simulink model "gm_sampleModel1427_5_sub"  (R2023a)
settings: Solver=VariableStepAuto  StartTime=0.0  StopTime=10.0  RelTol=1e-3
libraries: simulink x3
settings Model: Creator=user1  LastModifiedBy=user1
settings OptimizationCC: BlockReduction=off  ConditionallyExecuteInputs=off
settings DebuggingCC: InheritedTsInSrcMsg=none

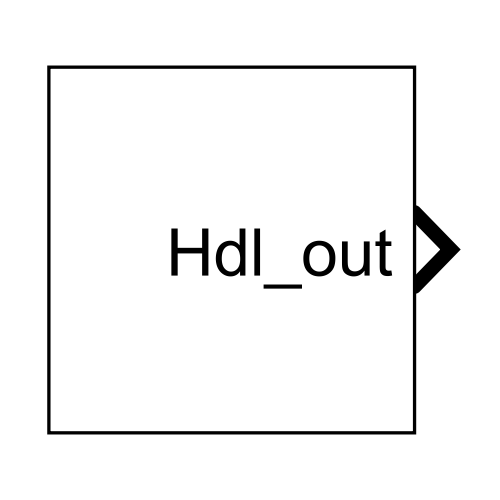
[thumbnail: Simulink's stored preview of the top-level diagram]
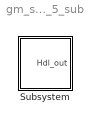
== system gm_sampleModel1427_5_sub ==
  Subsystem : Subsystem

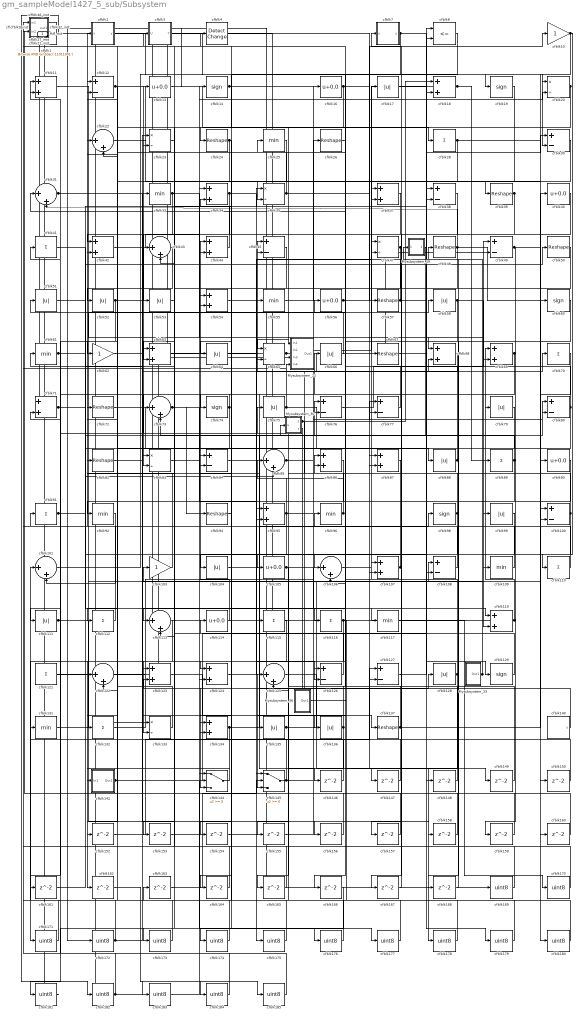
== system gm_sampleModel1427_5_sub/Subsystem ==
  Mysubsystem_19 : Subsystem
  Mysubsystem_22 : Subsystem
  Mysubsystem_30 : Subsystem
  Mysubsystem_33 : Subsystem
  Mysubsystem_36 : Subsystem
  cfblk1 : simulink/Logic and Bit Operations/Bitwise Operator  logicop=AND  UseBitMask=on  BitMask=bin2dec('11011001')  BitMaskRealWorld=Stored Integer
      settings: LibrarySourceBlock=|
      | hdlsllib/Logic and Bit
      | Operations/Bitwise
      | Operator
  cfblk10 : Gain  OutDataTypeStr=uint8
  cfblk{12,30,38,45,49,76..77,80,84,100,108,126..127} (13 alike) : Sum  Inputs=+-  OutDataTypeStr=uint8
  cfblk{22,31,43,73,85,101,106,113,122,125} (10 alike) : Sum  Inputs=|++  OutDataTypeStr=uint8
  cfblk102_inst : Subsystem
  cfblk103 : Gain  OutDataTypeStr=uint8
  cfblk{17,51..53,58,64,66,75,79,88,99,104,111,128,135..136} (16 alike) : Abs  OutDataTypeStr=uint8  SaturateOnIntegerOverflow=off
  cfblk{13,16,40,56,90,105,114} (7 alike) : Bias  Bias=0.0  SaturateOnIntegerOverflow=off
  cfblk{11,18,34,37,42,44,54,63,68..69,71,86..87,95,107,119,123..124,134} (19 alike) : Sum  OutDataTypeStr=uint8
  cfblk{25,33,55,61,92,96,109,117,131} (9 alike) : MinMax  OutDataTypeStr=uint8
  cfblk{28,41,70,89,91,110,112,115..116,121,132} (11 alike) : Sum  Inputs=+  OutDataTypeStr=uint8
  cfblk{14,19,60,74,98,129} (6 alike) : Signum
  cfblk130_inst : Subsystem
  cfblk{20,23,35,47,65,83,133} (7 alike) : Product  Inputs=*/  OutDataTypeStr=uint8  RndMeth=Zero  SaturateOnIntegerOverflow=on
  cfblk{24,26,39,48,50,57,67,72,82,94,137} (11 alike) : Reshape
  cfblk140 : Subsystem  mask(Counter Free-Running){NumBits=double(16), tsamp=double(-1)}
      mask prompts: NumBits "Simulink:masks:NumberOfBits_MP"; tsamp "Simulink:masks:SampleTime_MP"
      mask help: Simulink:masks:CounterFreeRunning_MD
  cfblk142 : Subsystem
  cfblk144 : Switch  OutDataTypeStr=uint8  SaturateOnIntegerOverflow=off  InputSameDT=off
  cfblk145 : Switch  OutDataTypeStr=uint8  SaturateOnIntegerOverflow=off  InputSameDT=off
  cfblk{146..150,152..168} (22 alike) : Delay  SampleTime=1
  cfblk{169..185} (17 alike) : DataTypeConversion  OutDataTypeStr=uint8  SaturateOnIntegerOverflow=off  RndMeth=Floor
  cfblk2 : Subsystem  mask(Compare To Constant){relop=<=, const=double(3), OutDataTypeStr=uint8, ZeroCross=on}
      mask prompts: relop "Simulink:masks:Operator_MP"; const "Simulink:masks:ConstantValue_MP"; OutDataTypeStr "Simulink:masks:OutputDataType_MP"; ZeroCross "Simulink:masks:EnableZerocrossingDetection_MP"
      mask help: Simulink:masks:CompareToConstant_MD
      mask init:
      | OutDataTypeStr = 'uint8';
      | ZeroCross = 'on';
      | blkName = 'sampleModel1427_5_sub/Subsystem/cfblk2';
      | const = double(3);
      | const_str = '3.0';
      | const_val = double(3);
      | relop = '<=';
      | setValue = 'fixdt(0, 8)';
      | str = '<= 3';
      mask TypeOptions relop: == | ~= | < | <= | >= | >
      mask TypeOptions OutDataTypeStr: Simulink:masks:uint8 | Simulink:masks:boolean
      mask Callback ZeroCross: sl('zeroCrossEnable', gcbh);
      mask Display: disp(str)
  cfblk21_inst : Subsystem
  cfblk27_inst : Subsystem
  cfblk3 : Subsystem  mask(Detect Rise Nonnegative){vinit=double(0), InputProcessing=Elements as channels (sample based), OutDataTypeStr=uint8}
      mask prompts: vinit "Simulink:masks:InitialCondition_MP"; InputProcessing "Simulink:masks:InputProcessing_MP"; OutDataTypeStr "Simulink:masks:OutputDataType_MP"
      mask help: Simulink:masks:DetectRiseNonnegative_MD
      mask init:
      | InputProcessing = 'Elements as channels (sample based)';
      | OutDataTypeStr = 'uint8';
      | vinit = double(0);
      mask TypeOptions InputProcessing: Simulink:masks:ColumnsAsChannelsFrameBased | Simulink:masks:ElementsAsChannelsSampleBased
      mask TypeOptions OutDataTypeStr: Simulink:masks:uint8 | Simulink:masks:boolean
      mask Display: fprintf('U >= 0\n&  NOT\nU/z >= 0')
  cfblk32_inst : Subsystem
  cfblk4 : simulink/Logic and Bit Operations/Detect Change  vinit=0  OutDataTypeStr=uint8
      settings: LibrarySourceBlock=|
      | hdlsllib/Logic and Bit
      | Operations/Detect
      | Change
  cfblk46_inst : Subsystem
  cfblk62 : Gain  OutDataTypeStr=uint8
  cfblk7 : Subsystem  mask(Compare To Constant){relop=<=, const=double(3), OutDataTypeStr=uint8, ZeroCross=on}
      mask prompts: relop "Simulink:masks:Operator_MP"; const "Simulink:masks:ConstantValue_MP"; OutDataTypeStr "Simulink:masks:OutputDataType_MP"; ZeroCross "Simulink:masks:EnableZerocrossingDetection_MP"
      mask help: Simulink:masks:CompareToConstant_MD
      mask init:
      | OutDataTypeStr = 'uint8';
      | ZeroCross = 'on';
      | blkName = 'sampleModel1427_5_sub/Subsystem/cfblk7';
      | const = double(3);
      | const_str = '3.0';
      | const_val = double(3);
      | relop = '<=';
      | setValue = 'fixdt(0, 8)';
      | str = '<= 3';
      mask TypeOptions relop: == | ~= | < | <= | >= | >
      mask TypeOptions OutDataTypeStr: Simulink:masks:uint8 | Simulink:masks:boolean
      mask Callback ZeroCross: sl('zeroCrossEnable', gcbh);
      mask Display: disp(str)
  cfblk8 : RelationalOperator  Operator=<=  OutDataTypeStr=boolean  InputSameDT=off
  cfblk9_inst : Subsystem
  Hdl_out : Outport  OutDataTypeStr=uint8  SampleTime=1
  wires:
  Mysubsystem_19/1(Out1) -> Mysubsystem_30/1(u)
  Mysubsystem_22/1(Out1) -> cfblk146/1
  Mysubsystem_30/1(Out1) -> cfblk18/1, cfblk144/3
  Mysubsystem_30/2(y) -> cfblk145/3
  Mysubsystem_33/1(Out1) -> cfblk103/1, Mysubsystem_19/1(In1)
  Mysubsystem_36/1(Out1) -> cfblk32_inst/2(in2)
  cfblk1/1 -> cfblk182/1
  cfblk10/1 -> cfblk30/2, cfblk110/1
  cfblk100/1 -> cfblk106/1, Mysubsystem_22/4(In4)
  cfblk101/1 -> cfblk19/1
  cfblk102_inst/1(out1) -> cfblk183/1
  cfblk103/1 -> cfblk2/1(u)
  cfblk104/1 -> cfblk96/1
  cfblk105/1 -> cfblk119/1, cfblk165/1
  cfblk106/1 -> cfblk17/1
  cfblk107/1 -> cfblk75/1, cfblk37/1
  cfblk108/1 -> cfblk32_inst/1(in1)
  cfblk109/1 -> cfblk67/1
  cfblk11/1 -> cfblk68/1
  cfblk110/1 -> cfblk12/1
  cfblk111/1 -> cfblk58/1, cfblk156/1
  cfblk112/1 -> cfblk42/2
  cfblk113/1 -> cfblk171/1
  cfblk114/1 -> cfblk44/1
  cfblk115/1 -> cfblk133/2
  cfblk116/1 -> cfblk163/1, cfblk162/1
  cfblk117/1 -> cfblk170/1
  cfblk119/1 -> cfblk69/1, Hdl_out/1
  cfblk12/1 -> cfblk39/1, cfblk152/1
  cfblk121/1 -> cfblk108/1
  cfblk122/1 -> cfblk80/1
  cfblk123/1 -> cfblk137/1
  cfblk124/1 -> cfblk56/1
  cfblk125/1 -> cfblk178/1
  cfblk126/1 -> cfblk82/1
  cfblk127/1 -> cfblk8/1
  cfblk128/1 -> cfblk130_inst/2(in2), cfblk166/1
  cfblk129/1 -> cfblk61/1
  cfblk13/1 -> cfblk28/1
  cfblk130_inst/1(out1) -> cfblk16/1
  cfblk131/1 -> cfblk76/1
  cfblk132/1 -> cfblk14/1
  cfblk133/1 -> cfblk51/1
  cfblk134/1 -> cfblk18/2, cfblk173/1, cfblk128/1
  cfblk135/1 -> cfblk66/1, cfblk100/1
  cfblk136/1 -> cfblk13/1, cfblk155/1, cfblk33/1
  cfblk137/1 -> cfblk40/1, cfblk34/2, cfblk114/1
  cfblk14/1 -> cfblk127/2, cfblk109/1
  cfblk140/1(y) -> cfblk123/2
  cfblk142/1(Out1) -> cfblk38/2, cfblk177/1
  cfblk144/1 -> cfblk142/1(In1)
  cfblk145/1 -> cfblk98/1, cfblk41/1
  cfblk146/1 -> cfblk101/1
  cfblk147/1 -> cfblk22/1
  cfblk148/1 -> cfblk86/1
  cfblk149/1 -> cfblk107/1
  cfblk150/1 -> cfblk71/2
  cfblk152/1 -> cfblk127/1
  cfblk153/1 -> cfblk124/2
  cfblk154/1 -> cfblk176/1
  cfblk155/1 -> cfblk8/2
  cfblk156/1 -> cfblk34/1
  cfblk157/1 -> cfblk144/2
  cfblk158/1 -> cfblk54/2
  cfblk159/1 -> cfblk45/1
  cfblk16/1 -> cfblk149/1, Mysubsystem_22/1(In1)
  cfblk160/1 -> cfblk12/2
  cfblk161/1 -> cfblk80/2
  cfblk162/1 -> cfblk185/1
  cfblk163/1 -> cfblk145/2
  cfblk164/1 -> cfblk43/2
  cfblk165/1 -> cfblk122/2
  cfblk166/1 -> cfblk181/1
  cfblk167/1 -> cfblk7/1(u)
  cfblk168/1 -> cfblk48/1
  cfblk169/1 -> cfblk46_inst/1(in1)
  cfblk17/1 -> cfblk20/1
  cfblk170/1 -> cfblk27_inst/1(in1)
  cfblk171/1 -> cfblk27_inst/2(in2)
  cfblk172/1 -> cfblk68/2, cfblk131/1
  cfblk173/1 -> cfblk9_inst/1(in1)
  cfblk174/1 -> cfblk9_inst/2(in2)
  cfblk175/1 -> cfblk72/1
  cfblk176/1 -> cfblk84/1
  cfblk177/1 -> cfblk84/2
  cfblk178/1 -> cfblk46_inst/2(in2)
  cfblk179/1 -> cfblk125/1
  cfblk18/1 -> Mysubsystem_22/2(In2), cfblk89/1
  cfblk180/1 -> cfblk125/2
  cfblk181/1 -> cfblk1/1
  cfblk182/1 -> cfblk184/1, cfblk91/1
  cfblk183/1 -> cfblk144/1
  cfblk184/1 -> cfblk102_inst/1(in1)
  cfblk185/1 -> cfblk102_inst/2(in2)
  cfblk19/1 -> cfblk124/1
  cfblk2/1(y) -> cfblk87/1
  cfblk20/1 -> cfblk63/2, cfblk22/2
  cfblk21_inst/1(out1) -> cfblk133/1, Mysubsystem_22/3(In3)
  cfblk22/1 -> cfblk180/1
  cfblk23/1 -> cfblk153/1
  cfblk24/1 -> cfblk134/2, cfblk122/1
  cfblk25/1 -> cfblk35/2
  cfblk26/1 -> cfblk136/1
  cfblk27_inst/1(out1) -> cfblk169/1
  cfblk28/1 -> cfblk90/1, cfblk52/1
  cfblk3/1(Y) -> cfblk150/1
  cfblk30/1 -> cfblk65/1
  cfblk31/1 -> cfblk37/2, cfblk134/1
  cfblk32_inst/1(out1) -> cfblk115/1
  cfblk33/1 -> cfblk69/2, cfblk42/1
  cfblk34/1 -> cfblk126/2, cfblk62/1
  cfblk35/1 -> cfblk77/2, cfblk21_inst/2(in2)
  cfblk37/1 -> cfblk53/1
  cfblk38/1 -> cfblk147/1
  cfblk39/1 -> cfblk64/1, cfblk47/1
  cfblk4/1 -> cfblk57/1
  cfblk40/1 -> cfblk105/1
  cfblk41/1 -> cfblk88/1
  cfblk42/1 -> cfblk44/2
  cfblk43/1 -> cfblk92/1
  cfblk44/1 -> cfblk23/2
  cfblk45/1 -> cfblk145/1
  cfblk46_inst/1(out1) -> cfblk71/1
  cfblk47/1 -> cfblk74/1, cfblk164/1
  cfblk48/1 -> cfblk60/1, cfblk31/2, cfblk135/1, cfblk104/1
  cfblk49/1 -> cfblk160/1, cfblk159/1
  cfblk50/1 -> cfblk113/2
  cfblk51/1 -> cfblk50/1
  cfblk52/1 -> cfblk111/1, cfblk158/1
  cfblk53/1 -> cfblk3/1(U)
  cfblk54/1 -> cfblk95/1
  cfblk55/1 -> cfblk26/1
  cfblk56/1 -> cfblk126/1, cfblk10/1
  cfblk57/1 -> cfblk45/2, cfblk179/1
  cfblk58/1 -> cfblk99/1, cfblk113/1
  cfblk60/1 -> cfblk168/1
  cfblk61/1 -> cfblk85/2, cfblk83/2
  cfblk62/1 -> cfblk43/1
  cfblk63/1 -> cfblk35/1
  cfblk64/1 -> cfblk47/2
  cfblk65/1 -> cfblk49/2, cfblk121/1
  cfblk66/1 -> cfblk11/1
  cfblk67/1 -> cfblk30/1
  cfblk68/1 -> cfblk65/2
  cfblk69/1 -> cfblk83/1, cfblk161/1
  cfblk7/1(y) -> cfblk129/1, cfblk106/2
  cfblk70/1 -> cfblk100/2
  cfblk71/1 -> cfblk38/1, cfblk107/2
  cfblk72/1 -> cfblk87/2
  cfblk73/1 -> cfblk95/2, cfblk94/1
  cfblk74/1 -> cfblk73/1, cfblk112/1
  cfblk75/1 -> cfblk130_inst/1(in1), cfblk148/1
  cfblk76/1 -> cfblk49/1
  cfblk77/1 -> cfblk21_inst/1(in1)
  cfblk79/1 -> cfblk167/1
  cfblk8/1 -> cfblk24/1
  cfblk80/1 -> cfblk31/1, cfblk123/1
  cfblk82/1 -> cfblk70/1
  cfblk83/1 -> cfblk20/2
  cfblk84/1 -> cfblk175/1
  cfblk85/1 -> cfblk79/1, cfblk76/2
  cfblk86/1 -> cfblk132/1
  cfblk87/1 -> cfblk86/2
  cfblk88/1 -> cfblk54/1, cfblk25/1
  cfblk89/1 -> cfblk73/2, cfblk119/2
  cfblk9_inst/1(out1) -> cfblk172/1
  cfblk90/1 -> cfblk174/1
  cfblk91/1 -> cfblk63/1, cfblk108/2, cfblk117/1
  cfblk92/1 -> cfblk101/2
  cfblk94/1 -> cfblk4/1
  cfblk95/1 -> cfblk77/1, cfblk154/1, cfblk55/1
  cfblk96/1 -> cfblk85/1, cfblk11/2
  cfblk98/1 -> cfblk23/1, cfblk116/1
  cfblk99/1 -> cfblk157/1

== system gm_sampleModel1427_5_sub/Subsystem/Mysubsystem_19 ==
  In1 : Inport  OutDataTypeStr=uint8  PortDimensions=1  SampleTime=1
  cfblk59 : Bias  Bias=0.0  SaturateOnIntegerOverflow=off
  Out1 : Outport  SampleTime=1
  wires:
  In1/1 -> cfblk59/1
  cfblk59/1 -> Out1/1

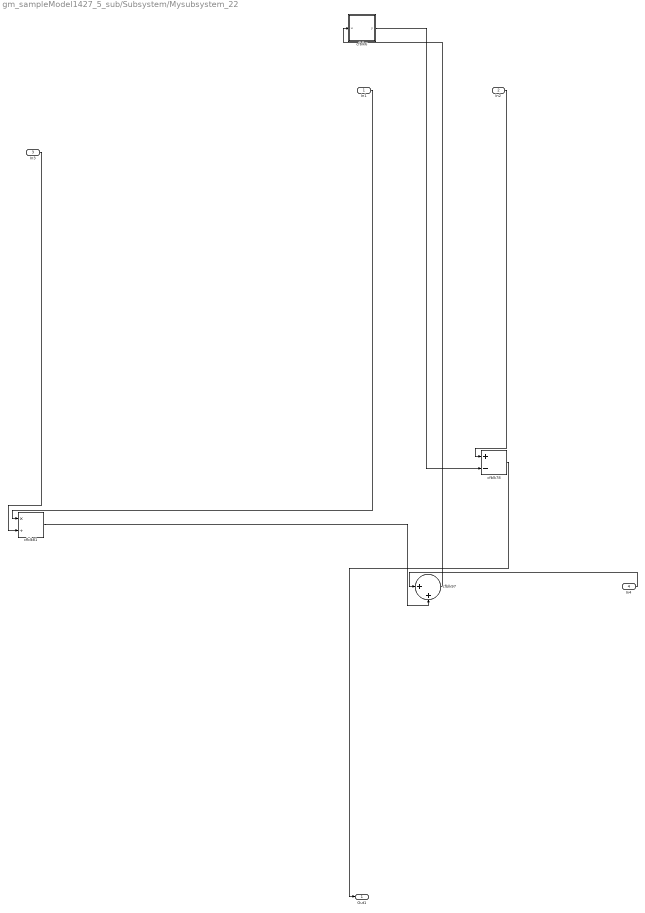
== system gm_sampleModel1427_5_sub/Subsystem/Mysubsystem_22 ==
  In1 : Inport  OutDataTypeStr=uint8  PortDimensions=1  SampleTime=1
  In2 : Inport  Port=2  OutDataTypeStr=uint8  PortDimensions=1  SampleTime=1
  In3 : Inport  Port=3  OutDataTypeStr=uint8  PortDimensions=1  SampleTime=1
  In4 : Inport  Port=4  OutDataTypeStr=uint8  PortDimensions=1  SampleTime=1
  cfblk6 : Subsystem  mask(Compare To Zero){relop=<=, OutDataTypeStr=boolean, ZeroCross=on}
      mask prompts: relop "Simulink:masks:Operator_MP"; OutDataTypeStr "Simulink:masks:OutputDataType_MP"; ZeroCross "Simulink:masks:EnableZerocrossingDetection_MP"
      mask help: Simulink:masks:CompareToZero_MD
      mask init:
      | OutDataTypeStr = 'boolean';
      | ZeroCross = 'on';
      | blkName = 'sampleModel1427_5_sub/Subsystem/Mysubsystem_22/cfblk6';
      | relop = '<=';
      | setValue = 'boolean';
      mask TypeOptions relop: == | ~= | < | <= | >= | >
      mask TypeOptions OutDataTypeStr: Simulink:masks:uint8 | Simulink:masks:boolean
      mask Callback ZeroCross: sl('zeroCrossEnable', gcbh);
      mask Display: disp([relop,' 0'])
  cfblk78 : Sum  Inputs=+-
  cfblk81 : Product  Inputs=*/  RndMeth=Zero  SaturateOnIntegerOverflow=on
  cfblk97 : Sum  Inputs=|++
  Out1 : Outport  SampleTime=1
  wires:
  In1/1 -> cfblk81/1
  In2/1 -> cfblk78/1
  In3/1 -> cfblk81/2
  In4/1 -> cfblk97/1
  cfblk6/1(y) -> cfblk78/2
  cfblk78/1 -> Out1/1
  cfblk81/1 -> cfblk97/2
  cfblk97/1 -> cfblk6/1(u)

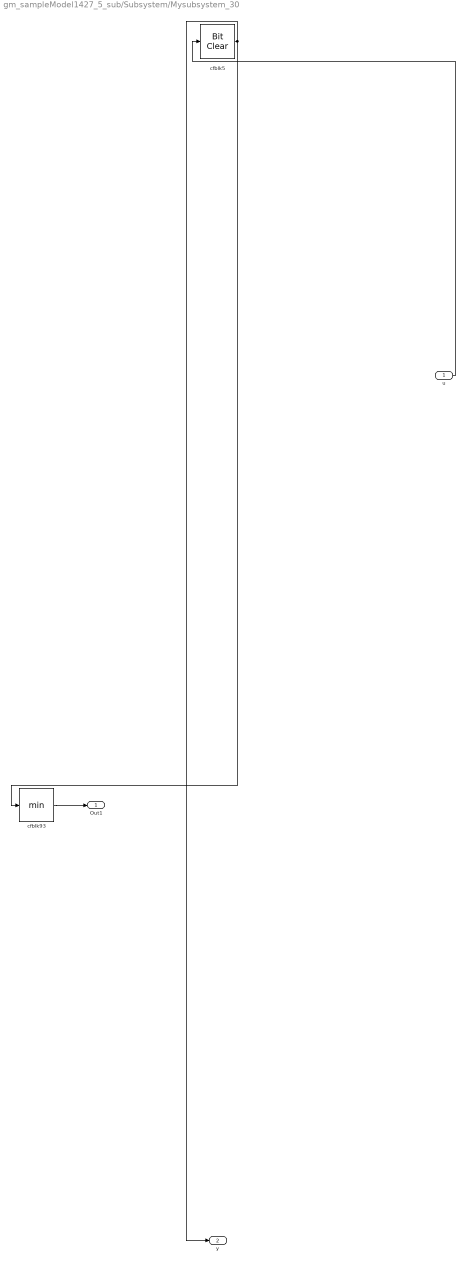
== system gm_sampleModel1427_5_sub/Subsystem/Mysubsystem_30 ==
  u : Inport  OutDataTypeStr=uint8  PortDimensions=1  SampleTime=1
  cfblk5 : simulink/Logic and Bit Operations/Bit Clear  iBit=0
      settings: LibrarySourceBlock=|
      | hdlsllib/Logic and Bit
      | Operations/Bit Clear
  cfblk93 : MinMax
  Out1 : Outport  SampleTime=1
  y : Outport  Port=2  SampleTime=1
  wires:
  u/1 -> cfblk5/1
  cfblk5/1 -> y/1, cfblk93/1
  cfblk93/1 -> Out1/1

== system gm_sampleModel1427_5_sub/Subsystem/Mysubsystem_33 ==
  cfblk118 : Sum  Inputs=+
  cfblk139 : Subsystem  mask(Counter Limited){uplimit=double(7), tsamp=double(-1)}
      mask prompts: uplimit "Simulink:masks:UpperLimit_MP"; tsamp "Simulink:masks:SampleTime_MP"
      mask help: Simulink:masks:CounterLimited_MD
      mask init:
      | nbits = double(8);
      | tsamp = double(-1);
      | uplimit = double(7);
  Out1 : Outport  SampleTime=1
  wires:
  cfblk118/1 -> Out1/1
  cfblk139/1(y) -> cfblk118/1

== system gm_sampleModel1427_5_sub/Subsystem/Mysubsystem_36 ==
  cfblk120 : Bias  Bias=0.0  SaturateOnIntegerOverflow=off
  cfblk141 : Ground
  Out1 : Outport  SampleTime=1
  wires:
  cfblk120/1 -> Out1/1
  cfblk141/1 -> cfblk120/1

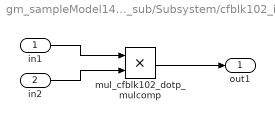
== system gm_sampleModel1427_5_sub/Subsystem/cfblk102_inst ==
  in1 : Inport  OutDataTypeStr=uint8  SampleTime=1
  in2 : Inport  Port=2  OutDataTypeStr=uint8  SampleTime=1
  mul_cfblk102_dotp_mulcomp : Product  Inputs=**  OutDataTypeStr=uint8  SampleTime=1
  out1 : Outport  OutDataTypeStr=uint8  SampleTime=1
  wires:
  in1/1 -> mul_cfblk102_dotp_mulcomp/1
  in2/1 -> mul_cfblk102_dotp_mulcomp/2
  mul_cfblk102_dotp_mulcomp/1 -> out1/1

== system gm_sampleModel1427_5_sub/Subsystem/cfblk130_inst ==
  in1 : Inport  OutDataTypeStr=uint8  SampleTime=1
  in2 : Inport  Port=2  OutDataTypeStr=uint8  SampleTime=1
  mul_cfblk130_dotp_mulcomp : Product  Inputs=**  OutDataTypeStr=uint8  SampleTime=1
  out1 : Outport  OutDataTypeStr=uint8  SampleTime=1
  wires:
  in1/1 -> mul_cfblk130_dotp_mulcomp/1
  in2/1 -> mul_cfblk130_dotp_mulcomp/2
  mul_cfblk130_dotp_mulcomp/1 -> out1/1

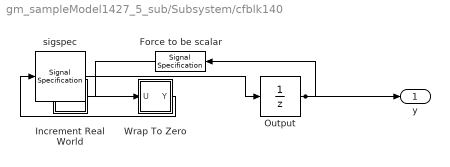
== system gm_sampleModel1427_5_sub/Subsystem/cfblk140 ==
  Force to be scalar : SignalSpecification  DisableCoverage=on  Dimensions=1
  Increment Real World : Subsystem  mask(Real World Value Increment){}
      mask help: Simulink:masks:RealWorldValueIncrement_MD
      mask Display: disp('V++')
  Output : UnitDelay  InitialCondition=0.0  SampleTime=tsamp  HasFrameUpgradeWarning=on
  Wrap To Zero : Subsystem  mask(Wrap To Zero){Threshold=double(65535)}
      mask prompts: Threshold "Simulink:masks:Threshold_MP"
      mask help: Simulink:masks:WrapToZero_MD
  sigspec : SignalSpecification  OutDataTypeStr=uint16  Dimensions=1
  y : Outport  SampleTime=1
  wires:
  Force to be scalar/1 -> Increment Real World/1(u)
  Increment Real World/1(y) -> Wrap To Zero/1(U)
  Output/1 -> Force to be scalar/1, y/1
  Wrap To Zero/1(Y) -> sigspec/1
  sigspec/1 -> Output/1

== system gm_sampleModel1427_5_sub/Subsystem/cfblk142 ==
  In1 : Inport  OutDataTypeStr=uint8  PortDimensions=1  SampleTime=1
  Out1 : Outport  SampleTime=1
  wires:
  In1/1 -> Out1/1

== system gm_sampleModel1427_5_sub/Subsystem/cfblk2 ==
  u : Inport  OutDataTypeStr=uint8  SampleTime=1
  Compare : RelationalOperator  Operator=<=  OutDataTypeStr=fixdt(0, 8)
  Constant : Constant  DisableCoverage=on  Value=const  OutDataTypeStr=Inherit: Inherit via back propagation  SampleTime=-1
  y : Outport  SampleTime=1
  wires:
  u/1 -> Compare/1
  Compare/1 -> y/1
  Constant/1 -> Compare/2

== system gm_sampleModel1427_5_sub/Subsystem/cfblk21_inst ==
  in1 : Inport  OutDataTypeStr=uint8  SampleTime=1
  in2 : Inport  Port=2  OutDataTypeStr=uint8  SampleTime=1
  mul_cfblk21_dotp_mulcomp : Product  Inputs=**  OutDataTypeStr=uint8  SampleTime=1
  out1 : Outport  OutDataTypeStr=uint8  SampleTime=1
  wires:
  in1/1 -> mul_cfblk21_dotp_mulcomp/1
  in2/1 -> mul_cfblk21_dotp_mulcomp/2
  mul_cfblk21_dotp_mulcomp/1 -> out1/1

== system gm_sampleModel1427_5_sub/Subsystem/cfblk27_inst ==
  in1 : Inport  OutDataTypeStr=uint8  SampleTime=1
  in2 : Inport  Port=2  OutDataTypeStr=uint8  SampleTime=1
  mul_cfblk27_dotp_mulcomp : Product  Inputs=**  OutDataTypeStr=uint8  SampleTime=1
  out1 : Outport  OutDataTypeStr=uint8  SampleTime=1
  wires:
  in1/1 -> mul_cfblk27_dotp_mulcomp/1
  in2/1 -> mul_cfblk27_dotp_mulcomp/2
  mul_cfblk27_dotp_mulcomp/1 -> out1/1

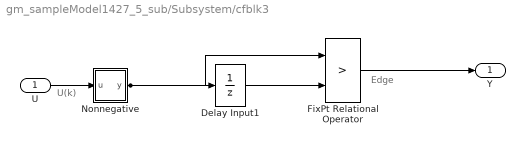
== system gm_sampleModel1427_5_sub/Subsystem/cfblk3 ==
  note: U(k)
  note: Edge
  U : Inport  OutDataTypeStr=uint8  SampleTime=1
  Delay Input1 : UnitDelay  Description=Store in Global RAM  DisableCoverage=on  InitialCondition=vinit  SampleTime=-1  HasFrameUpgradeWarning=on
  FixPt Relational Operator : RelationalOperator  Operator=>  OutDataTypeStr=fixdt(0, 8)  ZeroCross=off  InputSameDT=off
  Nonnegative : Subsystem  mask(Compare To Zero){relop=>=, OutDataTypeStr=boolean, ZeroCross=off}
      mask prompts: relop "Simulink:masks:Operator_MP"; OutDataTypeStr "Simulink:masks:OutputDataType_MP"; ZeroCross "Simulink:masks:EnableZerocrossingDetection_MP"
      mask help: Simulink:masks:CompareToZero_MD
      mask init:
      | OutDataTypeStr = 'boolean';
      | ZeroCross = 'off';
      | blkName = 'sampleModel1427_5_sub/Subsystem/cfblk3/Nonnegative';
      | relop = '>=';
      | setValue = 'boolean';
      mask TypeOptions relop: == | ~= | < | <= | >= | >
      mask TypeOptions OutDataTypeStr: Simulink:masks:uint8 | Simulink:masks:boolean
      mask Callback ZeroCross: sl('zeroCrossEnable', gcbh);
      mask Display: disp([relop,' 0'])
  Y : Outport  SampleTime=1
  wires:
  U/1 -> Nonnegative/1(u)
  Delay Input1/1 -> FixPt Relational Operator/2
  FixPt Relational Operator/1 -> Y/1
  Nonnegative/1(y) -> FixPt Relational Operator/1, Delay Input1/1

== system gm_sampleModel1427_5_sub/Subsystem/cfblk32_inst ==
  in1 : Inport  OutDataTypeStr=uint8  SampleTime=1
  in2 : Inport  Port=2  OutDataTypeStr=uint8  SampleTime=1
  mul_cfblk32_dotp_mulcomp : Product  Inputs=**  OutDataTypeStr=uint8  SampleTime=1
  out1 : Outport  OutDataTypeStr=uint8  SampleTime=1
  wires:
  in1/1 -> mul_cfblk32_dotp_mulcomp/1
  in2/1 -> mul_cfblk32_dotp_mulcomp/2
  mul_cfblk32_dotp_mulcomp/1 -> out1/1

== system gm_sampleModel1427_5_sub/Subsystem/cfblk46_inst ==
  in1 : Inport  OutDataTypeStr=uint8  SampleTime=1
  in2 : Inport  Port=2  OutDataTypeStr=uint8  SampleTime=1
  mul_cfblk46_dotp_mulcomp : Product  Inputs=**  OutDataTypeStr=uint8  SampleTime=1
  out1 : Outport  OutDataTypeStr=uint8  SampleTime=1
  wires:
  in1/1 -> mul_cfblk46_dotp_mulcomp/1
  in2/1 -> mul_cfblk46_dotp_mulcomp/2
  mul_cfblk46_dotp_mulcomp/1 -> out1/1

== system gm_sampleModel1427_5_sub/Subsystem/cfblk7 ==
  u : Inport  OutDataTypeStr=uint8  SampleTime=1
  Compare : RelationalOperator  Operator=<=  OutDataTypeStr=fixdt(0, 8)
  Constant : Constant  DisableCoverage=on  Value=const  OutDataTypeStr=Inherit: Inherit via back propagation  SampleTime=-1
  y : Outport  SampleTime=1
  wires:
  u/1 -> Compare/1
  Compare/1 -> y/1
  Constant/1 -> Compare/2

== system gm_sampleModel1427_5_sub/Subsystem/cfblk9_inst ==
  in1 : Inport  OutDataTypeStr=uint8  SampleTime=1
  in2 : Inport  Port=2  OutDataTypeStr=uint8  SampleTime=1
  mul_cfblk9_dotp_mulcomp : Product  Inputs=**  OutDataTypeStr=uint8  SampleTime=1
  out1 : Outport  OutDataTypeStr=uint8  SampleTime=1
  wires:
  in1/1 -> mul_cfblk9_dotp_mulcomp/1
  in2/1 -> mul_cfblk9_dotp_mulcomp/2
  mul_cfblk9_dotp_mulcomp/1 -> out1/1

== system gm_sampleModel1427_5_sub/Subsystem/Mysubsystem_22/cfblk6 ==
  u : Inport  OutDataTypeStr=uint8  SampleTime=1
  Compare : RelationalOperator  Operator=<=  OutDataTypeStr=boolean
  Constant : Constant  DisableCoverage=on  Value=0  OutDataTypeStr=Inherit: Inherit via back propagation  SampleTime=-1  PreserveConstantTs=on
  y : Outport  SampleTime=1
  wires:
  u/1 -> Compare/1
  Compare/1 -> y/1
  Constant/1 -> Compare/2

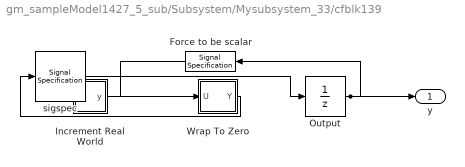
== system gm_sampleModel1427_5_sub/Subsystem/Mysubsystem_33/cfblk139 ==
  Force to be scalar : SignalSpecification  DisableCoverage=on  Dimensions=1
  Increment Real World : Subsystem  mask(Real World Value Increment){}
      mask help: Simulink:masks:RealWorldValueIncrement_MD
      mask Display: disp('V++')
  Output : UnitDelay  InitialCondition=0.0  SampleTime=tsamp  HasFrameUpgradeWarning=on
  Wrap To Zero : Subsystem  mask(Wrap To Zero){Threshold=double(7)}
      mask prompts: Threshold "Simulink:masks:Threshold_MP"
      mask help: Simulink:masks:WrapToZero_MD
  sigspec : SignalSpecification  OutDataTypeStr=uint8  Dimensions=1
  y : Outport  SampleTime=1
  wires:
  Force to be scalar/1 -> Increment Real World/1(u)
  Increment Real World/1(y) -> Wrap To Zero/1(U)
  Output/1 -> Force to be scalar/1, y/1
  Wrap To Zero/1(Y) -> sigspec/1
  sigspec/1 -> Output/1

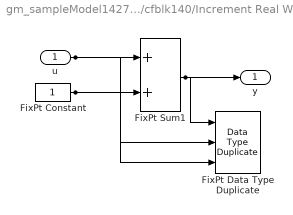
== system gm_sampleModel1427_5_sub/Subsystem/cfblk140/Increment Real World ==
  u : Inport  OutDataTypeStr=uint16  SampleTime=1
  FixPt Constant : Constant  DisableCoverage=on  OutDataTypeStr=Inherit: Inherit via back propagation  SampleTime=-1
  FixPt Data Type Duplicate : DataTypeDuplicate  DisableCoverage=on  NumInputPorts=3
  FixPt Sum1 : Sum  InputSameDT=on  OutDataTypeStr=Inherit: Inherit via back propagation  LockScale=on
  y : Outport  SampleTime=1
  wires:
  u/1 -> FixPt Sum1/1, FixPt Data Type Duplicate/2
  FixPt Constant/1 -> FixPt Sum1/2, FixPt Data Type Duplicate/3
  FixPt Sum1/1 -> FixPt Data Type Duplicate/1, y/1

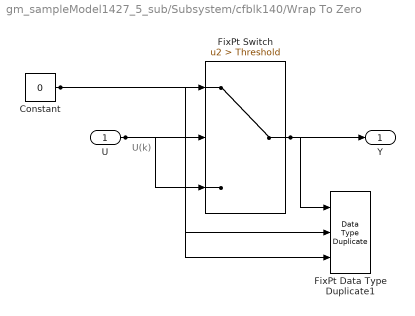
== system gm_sampleModel1427_5_sub/Subsystem/cfblk140/Wrap To Zero ==
  note: U(k)
  U : Inport  OutDataTypeStr=uint16  SampleTime=1
  Constant : Constant  DisableCoverage=on  Value=0  OutDataTypeStr=Inherit: Inherit via back propagation  SampleTime=-1
  FixPt Data Type Duplicate1 : DataTypeDuplicate  DisableCoverage=on  NumInputPorts=3
  FixPt Switch : Switch  Criteria=u2 > Threshold  Threshold=Threshold  OutDataTypeStr=Inherit: Inherit via back propagation  ZeroCross=off  SaturateOnIntegerOverflow=off  InputSameDT=off
  Y : Outport  SampleTime=1
  wires:
  U/1 -> FixPt Switch/3, FixPt Switch/2, FixPt Data Type Duplicate1/2
  Constant/1 -> FixPt Switch/1, FixPt Data Type Duplicate1/3
  FixPt Switch/1 -> FixPt Data Type Duplicate1/1, Y/1

== system gm_sampleModel1427_5_sub/Subsystem/cfblk3/Nonnegative ==
  u : Inport  OutDataTypeStr=uint8  SampleTime=1
  Compare : RelationalOperator  OutDataTypeStr=boolean  ZeroCross=off
  Constant : Constant  DisableCoverage=on  Value=0  OutDataTypeStr=Inherit: Inherit via back propagation  SampleTime=-1  PreserveConstantTs=on
  y : Outport  SampleTime=1
  wires:
  u/1 -> Compare/1
  Compare/1 -> y/1
  Constant/1 -> Compare/2

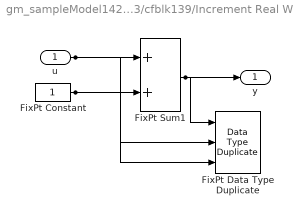
== system gm_sampleModel1427_5_sub/Subsystem/Mysubsystem_33/cfblk139/Increment Real World ==
  u : Inport  OutDataTypeStr=uint8  SampleTime=1
  FixPt Constant : Constant  DisableCoverage=on  OutDataTypeStr=Inherit: Inherit via back propagation  SampleTime=-1
  FixPt Data Type Duplicate : DataTypeDuplicate  DisableCoverage=on  NumInputPorts=3
  FixPt Sum1 : Sum  InputSameDT=on  OutDataTypeStr=Inherit: Inherit via back propagation  LockScale=on
  y : Outport  SampleTime=1
  wires:
  u/1 -> FixPt Sum1/1, FixPt Data Type Duplicate/2
  FixPt Constant/1 -> FixPt Sum1/2, FixPt Data Type Duplicate/3
  FixPt Sum1/1 -> FixPt Data Type Duplicate/1, y/1

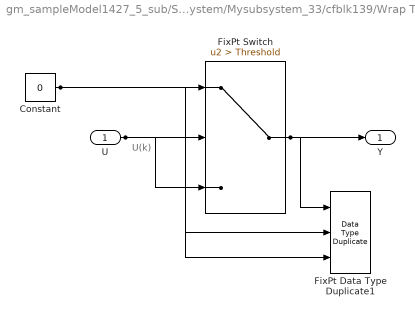
== system gm_sampleModel1427_5_sub/Subsystem/Mysubsystem_33/cfblk139/Wrap To Zero ==
  note: U(k)
  U : Inport  OutDataTypeStr=uint8  SampleTime=1
  Constant : Constant  DisableCoverage=on  Value=0  OutDataTypeStr=Inherit: Inherit via back propagation  SampleTime=-1
  FixPt Data Type Duplicate1 : DataTypeDuplicate  DisableCoverage=on  NumInputPorts=3
  FixPt Switch : Switch  Criteria=u2 > Threshold  Threshold=Threshold  OutDataTypeStr=Inherit: Inherit via back propagation  ZeroCross=off  SaturateOnIntegerOverflow=off  InputSameDT=off
  Y : Outport  SampleTime=1
  wires:
  U/1 -> FixPt Switch/3, FixPt Switch/2, FixPt Data Type Duplicate1/2
  Constant/1 -> FixPt Switch/1, FixPt Data Type Duplicate1/3
  FixPt Switch/1 -> FixPt Data Type Duplicate1/1, Y/1
